simulink model "a3"  (Simulink 8.7)
settings: Solver=VariableStepAuto  StartTime=0.0  StopTime=10.0  RelTol=1e-3
settings Model: Creator=birger  LastModifiedBy=birger
settings DataIOCC: LimitDataPoints=off  SaveFormat=Dataset
settings DebuggingCC: UnderspecifiedInitializationDetection=Simplified  MergeDetectMultiDrivingBlocksExec=error
settings HardwareCC: ProdBitPerPointer=64  ProdLargestAtomicFloat=Float  ProdIntDivRoundTo=Zero  ProdEndianess=LittleEndian  ProdWordSize=64  ProdHWDeviceType=Intel->x86-64 (Windows64)
settings ModelReferenceCC: PropagateSignalLabelsOutOfModel=on
settings ConfigComp: CovModelRefEnable=off

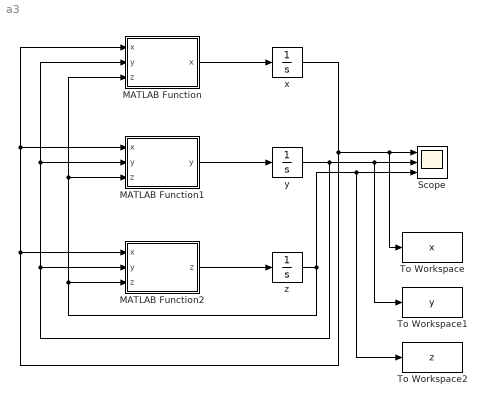
== system a3 ==
  MATLAB Function : MATLAB Function  TreatAsAtomicUnit=on
  MATLAB Function1 : MATLAB Function  TreatAsAtomicUnit=on
  MATLAB Function2 : MATLAB Function  TreatAsAtomicUnit=on
  Scope : Scope  NumInputPorts=3
  To Workspace : ToWorkspace  VariableName=x  SaveFormat=Timeseries  SampleTime=-1
  To Workspace1 : ToWorkspace  VariableName=y  SaveFormat=Timeseries  SampleTime=-1
  To Workspace2 : ToWorkspace  VariableName=z  SaveFormat=Timeseries  SampleTime=-1
  x : Integrator  InitialCondition=0.01
  y : Integrator  InitialCondition=0.01
  z : Integrator
  wires:
  x/1 -> To Workspace/1, Scope/1, MATLAB Function2/1(x), MATLAB Function1/1(x), MATLAB Function/1("x ")
  y/1 -> MATLAB Function2/2(y), MATLAB Function1/2("y "), MATLAB Function/2(y), To Workspace1/1, Scope/2
  z/1 -> MATLAB Function2/3("z "), MATLAB Function1/3(z), MATLAB Function/3(z), To Workspace2/1, Scope/3
  MATLAB Function/1(x) -> x/1
  MATLAB Function1/1(y) -> y/1
  MATLAB Function2/1(z) -> z/1

== matlab function MATLAB Function1 ==
  data: x input double; y output double; y input double; z input double
function y = fcn(x,y,z)
%#codegen

y = (40 -z) * x - y;

== matlab function MATLAB Function ==
  data: x input double; x output double; y input double; z input double
function x = fcn(x,y,z)
%#codegen

x = -10 * (x-y);

== matlab function MATLAB Function2 ==
  data: x input double; z output double; y input double; z input double
function z = fcn(x,y,z)
%#codegen

z = x * y - 2.67 * z;
